simulink model "simexexa21"  (Simulink 2.09)
settings: Solver=ode45  StartTime=0.0  StopTime=100.0  RelTol=1e-3  AbsTol=1e-6
libraries: simulink x1
settings Model: ConsistencyChecking=off  RTWTemplateMakefile=grt_vc.tmf

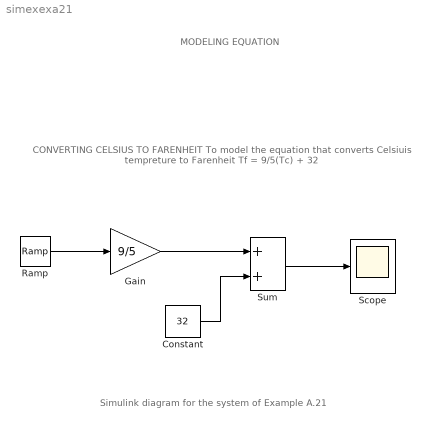
== system simexexa21 ==
  note: Simulink diagram for the system of Example A.21
  note: CONVERTING CELSIUS TO FARENHEIT
      |
      | To model the equation that converts Celsiuis tempreture to Farenheit
      |
      | Tf = 9/5(Tc) + 32
  note: MODELING EQUATION
  Constant : Constant  Value=32
  Gain : Gain  Gain=9/5
  Ramp : simulink/Sources/Ramp  slope=1  start=0  X0=0
  Scope : Scope
      settings: TickLabels=on  TimeRange=auto  YMin=-5  YMax=5  SaveToWorkspace=off  SaveName=ScopeData
  Sum : Sum  Inputs=++
  wires:
  Ramp/1 -> Gain/1
  Gain/1 -> Sum/1
  Sum/1 -> Scope/1
  Constant/1 -> Sum/2
